simulink model "AirCooledDataCenterTemperatureProfile"  (R2025b)
settings: Solver=daessc  StartTime=0.0  StopTime=24*3600  MaxStep=1  RelTol=1e-3  AbsTol=1e-3
PreLoadFcn:
  | if ~exist("airCooledDataCenter")
  |     setModelParam;
  | end
undefined symbols (not defined in the file or in its folder): airCooledDataCenter, DiscIntNeverNeededParam, value
libraries: fl_lib x166, nesl_utility x25, datacenter_lib x24, simulink_extras x9
(part 4 of 4)

== system AirCooledDataCenterTemperatureProfile/DataCenter/Air Cooled PDU Assembly 3/Rack Air Cooling/dT ==
  Cold : fl_lib/Thermal/Thermal Sensors/Temperature Sensor  temperature_measure=foundation.enum.MeasurementReference.absolute
      settings: InternalSimscapePortConfiguration="{\"Bottom\":[],\"Left\":[{\"id\":\"A\",\"label\":\"A\",\"type\":\"foundation.thermal.thermal\"}],\"Right\":[{\"id\":\"T\",\"label\":\"T\",\"type\":\"output\"}],\"Top\":[]}"
  Hot : fl_lib/Thermal/Thermal Sensors/Temperature Sensor  temperature_measure=foundation.enum.MeasurementReference.absolute
      settings: InternalSimscapePortConfiguration="{\"Bottom\":[],\"Left\":[{\"id\":\"A\",\"label\":\"A\",\"type\":\"foundation.thermal.thermal\"}],\"Right\":[{\"id\":\"T\",\"label\":\"T\",\"type\":\"output\"}],\"Top\":[]}"
  PS Subtract : fl_lib/Physical Signals/Functions/PS Subtract
  C : PMIOPort  Side=Left
  H : PMIOPort  Port=2  Side=Right
  dT : PMIOPort  Port=3  Side=Right
  connections:
  Cold/LConn1 -- C/RConn1
  dT/RConn1 -- PS Subtract/RConn1
  PS Subtract/LConn1 -- Cold/RConn1
  PS Subtract/LConn2 -- Hot/RConn1
  Hot/LConn1 -- H/RConn1

== system AirCooledDataCenterTemperatureProfile/DataCenter/Air Cooled PDU Assembly 3/Rack Air Cooling/m_dot_Cp ==
  Fluid Density : fl_lib/Physical Signals/Sources/PS Constant  constant=fluidDen kg/m^3
  Fluid Sp. Heat : fl_lib/Physical Signals/Sources/PS Constant  constant=fluidCp J/(K*kg)
  PS Product3 : fl_lib/Physical Signals/Functions/PS Product
  PS Product4 : fl_lib/Physical Signals/Functions/PS Product
  " " : PMIOPort  Side=Left
  m : PMIOPort  Port=2  Side=Right
  connections:
  PS Product4/LConn2 -- PS Product3/RConn1
  Fluid Density/RConn1 -- PS Product3/LConn1
  PS Product3/LConn2 -- m/RConn1
  PS Product4/LConn1 -- Fluid Sp. Heat/RConn1
  PS Product4/RConn1 -- " "/RConn1

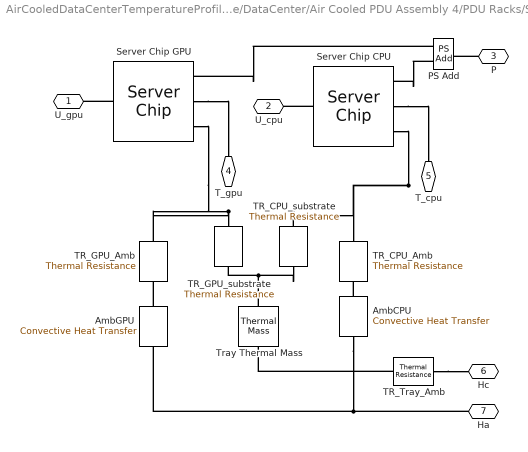
== system AirCooledDataCenterTemperatureProfile/DataCenter/Air Cooled PDU Assembly 4/PDU Racks/Server Tray ==
  AmbCPU : fl_lib/Thermal/Thermal Elements/Convective Heat Transfer  thermal_type=foundation.enum.constant_variable.constant  area=cpuSurfArea*nCPU m^2  heat_tr_coeff=htc W/(K*m^2)  min_heat_tr_coeff=1e-3 W/(K*m^2)  T_specify=off  T_priority=None  T=0 K  T_nominal_specify=off  T_nominal_value=1  T_nominal_unit=K  Q_specify=off  Q_priority=None  Q=0 W  Q_nominal_specify=off  Q_nominal_value=1  Q_nominal_unit=W
  AmbGPU : fl_lib/Thermal/Thermal Elements/Convective Heat Transfer  thermal_type=foundation.enum.constant_variable.constant  area=gpuSurfArea*nGPU m^2  heat_tr_coeff=htc W/(K*m^2)  min_heat_tr_coeff=1e-3 W/(K*m^2)  T_specify=off  T_priority=None  T=0 K  T_nominal_specify=off  T_nominal_value=1  T_nominal_unit=K  Q_specify=off  Q_priority=None  Q=0 W  Q_nominal_specify=off  Q_nominal_value=1  Q_nominal_unit=W
  PS Add : fl_lib/Physical Signals/Functions/PS Add
  Server Chip CPU : datacenter_lib/Server Chip  processorType=ProcessorType.CPU  numGPUs=4  numCPUs=nCPU  gpuTDP=1200 W  gpuIdlePower=300 W  gpuPowerExponent=1.4  hbmPowPerGPU=80 W  hbmUtilizationFrac=0.7  cpuTDP=cpuTDPperSocket W  cpuIdlePower=cpuIdlePower W  cpuPowerExponent=cpuExponent  PleakageCoeff=cpuLeakage W/K  chipTnominal=cpuNominalDieT K  chipCth=cpuDieThermalC J/K  T_specify=on  T_priority=High  T=initialT K  T_nominal_specify=off  T_nominal_value=1  T_nominal_unit=K  Q_specify=off  Q_priority=None  Q=0 W  Q_nominal_specify=off  Q_nominal_value=1  Q_nominal_unit=W
      settings: InternalSimscapePortConfiguration="{\"Bottom\":[{\"id\":\"H\",\"label\":\"H\",\"type\":\"foundation.thermal.thermal\"}],\"Left\":[{\"id\":\"U\",\"label\":\"U\",\"type\":\"input\"}],\"Right\":[{\"id\":\"Pow\",\"label\":\"P\",\"type\":\"output\"},{\"id\":\"Tchip\",\"label\":\"T\",\"type\":\"output\"}],\"Top\":[]}"
  Server Chip GPU : datacenter_lib/Server Chip  processorType=ProcessorType.GPU  numGPUs=nGPU  numCPUs=nCPU  gpuTDP=gpuTDPperDie W  gpuIdlePower=gpuIdlePower W  gpuPowerExponent=gpuExponent  hbmPowPerGPU=gpuHBMpower W  hbmUtilizationFrac=gpuHBMutil  cpuTDP=cpuTDPperSocket W  cpuIdlePower=cpuIdlePower W  cpuPowerExponent=1.1  PleakageCoeff=gpuLeakage W/K  chipTnominal=gpuNominalDieT K  chipCth=gpuDieThermalC J/K  T_specify=on  T_priority=High  T=initialT K  T_nominal_specify=off  T_nominal_value=1  T_nominal_unit=K  Q_specify=off  Q_priority=None  Q=0 W  Q_nominal_specify=off  Q_nominal_value=1  Q_nominal_unit=W
      settings: InternalSimscapePortConfiguration="{\"Bottom\":[{\"id\":\"H\",\"label\":\"H\",\"type\":\"foundation.thermal.thermal\"}],\"Left\":[{\"id\":\"U\",\"label\":\"U\",\"type\":\"input\"}],\"Right\":[{\"id\":\"Pow\",\"label\":\"P\",\"type\":\"output\"},{\"id\":\"Tchip\",\"label\":\"T\",\"type\":\"output\"}],\"Top\":[]}"
  TR_CPU_Amb : fl_lib/Thermal/Thermal Elements/Thermal Resistance  resistance=cpuAmbientR/nCPU K/W  T_specify=off  T_priority=None  T=0 K  T_nominal_specify=off  T_nominal_value=1  T_nominal_unit=K  Q_specify=off  Q_priority=None  Q=0 W  Q_nominal_specify=off  Q_nominal_value=1  Q_nominal_unit=W
  TR_CPU_substrate : fl_lib/Thermal/Thermal Elements/Thermal Resistance  resistance=cpuHeatSinkR/nCPU K/W  T_specify=off  T_priority=None  T=0 K  T_nominal_specify=off  T_nominal_value=1  T_nominal_unit=K  Q_specify=off  Q_priority=None  Q=0 W  Q_nominal_specify=off  Q_nominal_value=1  Q_nominal_unit=W
  TR_GPU_Amb : fl_lib/Thermal/Thermal Elements/Thermal Resistance  resistance=gpuAmbientR/nGPU K/W  T_specify=off  T_priority=None  T=0 K  T_nominal_specify=off  T_nominal_value=1  T_nominal_unit=K  Q_specify=off  Q_priority=None  Q=0 W  Q_nominal_specify=off  Q_nominal_value=1  Q_nominal_unit=W
  TR_GPU_substrate : fl_lib/Thermal/Thermal Elements/Thermal Resistance  resistance=gpuHeatSinkR/nGPU K/W  T_specify=off  T_priority=None  T=0 K  T_nominal_specify=off  T_nominal_value=1  T_nominal_unit=K  Q_specify=off  Q_priority=None  Q=0 W  Q_nominal_specify=off  Q_nominal_value=1  Q_nominal_unit=W
  TR_Tray_Amb : fl_lib/Thermal/Thermal Elements/Thermal Resistance  resistance=trayThermalR K/W  T_specify=off  T_priority=None  T=0 K  T_nominal_specify=off  T_nominal_value=1  T_nominal_unit=K  Q_specify=off  Q_priority=None  Q=0 W  Q_nominal_specify=off  Q_nominal_value=1  Q_nominal_unit=W
  Tray Thermal Mass : fl_lib/Thermal/Thermal Elements/Thermal Mass  mass_type=foundation.enum.constant_variable.constant  mass=trayMass kg  sp_heat=trayCp J/(K*kg)  mass_min=1e-6 kg  num_ports=foundation.enum.numPorts2.two  m_specify=off  m_priority=High  m=1 kg  m_nominal_specify=off  m_nominal_value=1  m_nominal_unit=kg  T_specify=on  T_priority=High  T=initialT K  T_nominal_specify=off  T_nominal_value=1  T_nominal_unit=K  Q_specify=off  Q_priority=None  Q=0 W  Q_nominal_specify=off  Q_nominal_value=1  Q_nominal_unit=W
      settings: InternalSimscapePortConfiguration="{\"Bottom\":[],\"Left\":[{\"id\":\"M\",\"label\":\"\",\"type\":\"foundation.thermal.thermal\"}],\"Right\":[{\"id\":\"N\",\"label\":\"\",\"type\":\"foundation.thermal.thermal\"}],\"Top\":[]}"
  U_gpu : PMIOPort  Side=Left
  U_cpu : PMIOPort  Port=2  Side=Left
  P : PMIOPort  Port=3  Side=Right
  T_gpu : PMIOPort  Port=4  Side=Right
  T_cpu : PMIOPort  Port=5  Side=Right
  Hc : PMIOPort  Port=6  Side=Right
  Ha : PMIOPort  Port=7  Side=Left
  connections:
  AmbCPU/LConn1 -- TR_CPU_Amb/RConn1
  PS Add/LConn2 -- Server Chip CPU/RConn1
  PS Add/LConn1 -- Server Chip GPU/RConn1
  P/RConn1 -- PS Add/RConn1
  Ha/RConn1 -- AmbGPU/RConn1 -- AmbCPU/RConn1
  AmbGPU/LConn1 -- TR_GPU_Amb/LConn1
  TR_Tray_Amb/RConn1 -- Hc/RConn1
  Server Chip CPU/RConn2 -- T_cpu/RConn1
  Server Chip CPU/LConn1 -- U_cpu/RConn1
  Server Chip GPU/LConn1 -- U_gpu/RConn1
  TR_Tray_Amb/LConn1 -- Tray Thermal Mass/RConn1
  TR_GPU_substrate/LConn1 -- Server Chip GPU/RConn3 -- TR_GPU_Amb/RConn1
  Server Chip CPU/RConn3 -- TR_CPU_Amb/LConn1 -- TR_CPU_substrate/LConn1
  Server Chip GPU/RConn2 -- T_gpu/RConn1
  TR_CPU_substrate/RConn1 -- TR_GPU_substrate/RConn1 -- Tray Thermal Mass/LConn1

== system AirCooledDataCenterTemperatureProfile/DataCenter/Air Cooled PDU Assembly 4/Rack Air Cooling/Q ==
  Controlled Heat Flow Rate Source : fl_lib/Thermal/Thermal Sources/Controlled Heat Flow Rate Source
  PS Product2 : fl_lib/Physical Signals/Functions/PS Product
  Thermal Reference : fl_lib/Thermal/Thermal Elements/Thermal Reference
  dT : PMIOPort  Side=Left
  m.Cp : PMIOPort  Port=2  Side=Left
  Q : PMIOPort  Port=3  Side=Right
  connections:
  PS Product2/RConn1 -- Controlled Heat Flow Rate Source/RConn1
  Thermal Reference/LConn1 -- Controlled Heat Flow Rate Source/RConn2
  PS Product2/LConn1 -- dT/RConn1
  Controlled Heat Flow Rate Source/LConn1 -- Q/RConn1
  m.Cp/RConn1 -- PS Product2/LConn2

== system AirCooledDataCenterTemperatureProfile/DataCenter/Air Cooled PDU Assembly 4/Rack Air Cooling/dT ==
  Cold : fl_lib/Thermal/Thermal Sensors/Temperature Sensor  temperature_measure=foundation.enum.MeasurementReference.absolute
      settings: InternalSimscapePortConfiguration="{\"Bottom\":[],\"Left\":[{\"id\":\"A\",\"label\":\"A\",\"type\":\"foundation.thermal.thermal\"}],\"Right\":[{\"id\":\"T\",\"label\":\"T\",\"type\":\"output\"}],\"Top\":[]}"
  Hot : fl_lib/Thermal/Thermal Sensors/Temperature Sensor  temperature_measure=foundation.enum.MeasurementReference.absolute
      settings: InternalSimscapePortConfiguration="{\"Bottom\":[],\"Left\":[{\"id\":\"A\",\"label\":\"A\",\"type\":\"foundation.thermal.thermal\"}],\"Right\":[{\"id\":\"T\",\"label\":\"T\",\"type\":\"output\"}],\"Top\":[]}"
  PS Subtract : fl_lib/Physical Signals/Functions/PS Subtract
  C : PMIOPort  Side=Left
  H : PMIOPort  Port=2  Side=Right
  dT : PMIOPort  Port=3  Side=Right
  connections:
  Cold/LConn1 -- C/RConn1
  dT/RConn1 -- PS Subtract/RConn1
  PS Subtract/LConn1 -- Cold/RConn1
  PS Subtract/LConn2 -- Hot/RConn1
  Hot/LConn1 -- H/RConn1

== system AirCooledDataCenterTemperatureProfile/DataCenter/Air Cooled PDU Assembly 4/Rack Air Cooling/m_dot_Cp ==
  Fluid Density : fl_lib/Physical Signals/Sources/PS Constant  constant=fluidDen kg/m^3
  Fluid Sp. Heat : fl_lib/Physical Signals/Sources/PS Constant  constant=fluidCp J/(K*kg)
  PS Product3 : fl_lib/Physical Signals/Functions/PS Product
  PS Product4 : fl_lib/Physical Signals/Functions/PS Product
  " " : PMIOPort  Side=Left
  m : PMIOPort  Port=2  Side=Right
  connections:
  PS Product4/LConn2 -- PS Product3/RConn1
  Fluid Density/RConn1 -- PS Product3/LConn1
  PS Product3/LConn2 -- m/RConn1
  PS Product4/LConn1 -- Fluid Sp. Heat/RConn1
  PS Product4/RConn1 -- " "/RConn1
